simulink model "part2"  (R2015a)
settings: Solver=ode45  StartTime=0.0  StopTime=10.0  RelTol=1e-3
libraries: simulink x1
settings Model: Creator=vdrouinv  LastModifiedBy=vdrouinv

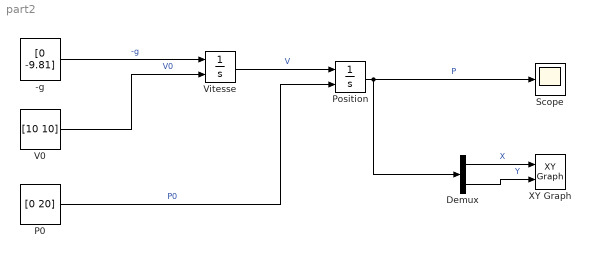
== system part2 ==
  -g : Constant  Value=[0 -9.81]
  Demux : Demux  Outputs=2
  P0 : Constant  Value=[0 20]
  Position : Integrator  InitialConditionSource=external
  Scope : Scope
  V0 : Constant  Value=[10 10]
  Vitesse : Integrator  InitialConditionSource=external
  XY Graph : simulink/Sinks/XY Graph  xmin=0  xmax=100  ymin=-400  ymax=50  st=-1
  wires:
  -g/1 -> Vitesse/1  "-g"
  V0/1 -> Vitesse/2  "V0"
  P0/1 -> Position/2  "P0"
  Vitesse/1 -> Position/1  "V"
  Position/1 -> Demux/1, Scope/1  "P"
  Demux/1 -> XY Graph/1  "X"
  Demux/2 -> XY Graph/2  "Y"
